simulink model "lab1dulepovMinina22017"  (R2017a)
settings: Solver=ode23tb  StartTime=0.0  StopTime=1  MaxStep=1e-4  RelTol=1e-5
undefined symbols (not defined in the file): load, source, transparam
libraries: powerlib x9, powerlib_meascontrol x3
settings Model: Creator=Student11  LastModifiedBy=админ
settings SolverCC: MaxConsecutiveMinStep=2
settings DebuggingCC: IgnoredZcDiagnostic=none  UnconnectedInputMsg=none  UnconnectedOutputMsg=none  UnconnectedLineMsg=none
settings SimscapeCC: SimscapeNormalizeSystem=off

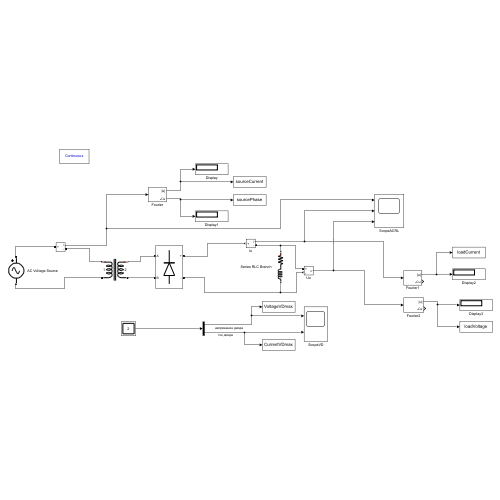
[thumbnail: Simulink's stored preview of the top-level diagram]
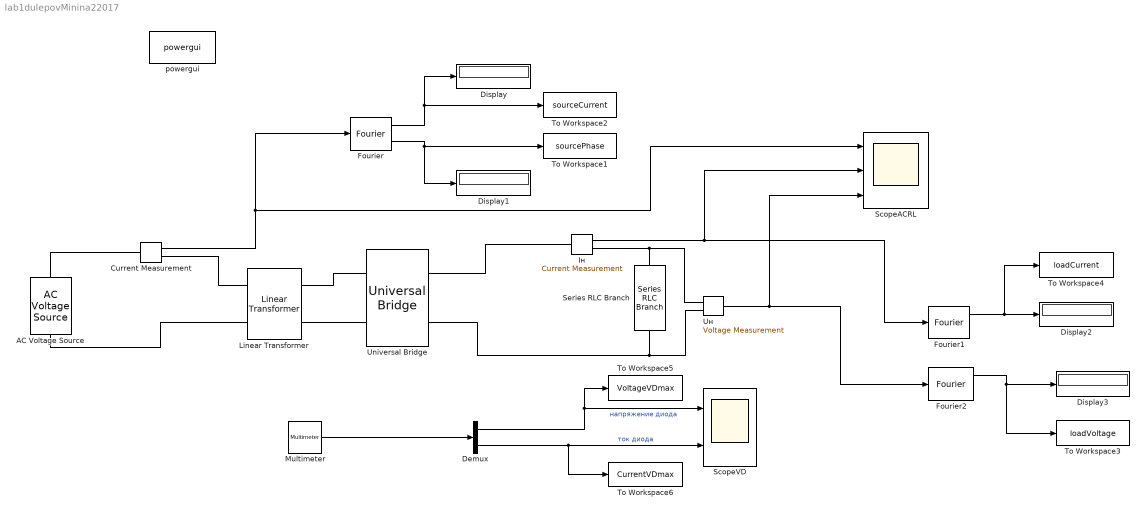
== system lab1dulepovMinina22017 ==
  AC Voltage Source : powerlib/Electrical Sources/AC Voltage Source  Amplitude=source.voltage  Phase=0  Frequency=source.freq  SampleTime=0  Measurements=None  BusType=swing  Pref=10e3  Qref=0  Qmin=-inf  Qmax=+inf
  Current Measurement : powerlib/Measurements/Current Measurement  PhasorSimulation=off  OutputType=Complex  PSBequivalent=0
  Demux : Demux  Outputs=2
  Display{,1..3} (4 alike) : Display
  Fourier : powerlib_meascontrol/Measurements/Fourier  Freq=source.freq  n=1  InInit=[0, 0]  Ts=0
  Fourier1 : powerlib_meascontrol/Measurements/Fourier  Freq=source.freq  n=0  InInit=[0, 0]  Ts=0
  Fourier2 : powerlib_meascontrol/Measurements/Fourier  Freq=source.freq  n=0  InInit=[0, 0]  Ts=0
  Iн : powerlib/Measurements/Current Measurement  PhasorSimulation=off  OutputType=Complex  PSBequivalent=0
  Linear Transformer : powerlib/Elements/Linear Transformer  UNITS=SI  NominalPower=[transparam.power source.freq]  winding1=[transparam.volt1wing 0.01 0.000001]  winding2=[transparam.volt2wing 0.04 0.000004]  ThreeWindings=off  winding3=[3.15e+05 992.25 63.169]  RmLm=[5000 5000]  Measurements=None  DataType=on
  Multimeter : powerlib/Measurements/Multimeter  L=10  sel=[1 7]  yselected={}  Gain=[1 1]  OutputType=Complex  PlotAtSimulationStop=off  PhasorSimulation=off
  ScopeVD : Scope  NumInputPorts=2
  ScopeАСRL : Scope  NumInputPorts=3
  Series RLC Branch : powerlib/Elements/Series RLC Branch  LConnTagsString=__new0  RConnTagsString=__new0  BranchType=RL  Resistance=load.Res  Inductance=load.Ind  SetiL0=off  InitialCurrent=0  Capacitance=1e-6  Setx0=off  InitialVoltage=0  Measurements=None
  To Workspace1 : ToWorkspace  VariableName=sourcePhase  SampleTime=-1
      settings: Save2DSignal=2-D array (concatenate along first dimension)
  To Workspace2 : ToWorkspace  VariableName=sourceCurrent  SampleTime=-1
      settings: Save2DSignal=2-D array (concatenate along first dimension)
  To Workspace3 : ToWorkspace  VariableName=loadVoltage  SampleTime=-1
      settings: Save2DSignal=2-D array (concatenate along first dimension)
  To Workspace4 : ToWorkspace  VariableName=loadCurrent  SampleTime=-1
      settings: Save2DSignal=2-D array (concatenate along first dimension)
  To Workspace5 : ToWorkspace  VariableName=VoltageVDmax  SampleTime=-1
      settings: Save2DSignal=2-D array (concatenate along first dimension)
  To Workspace6 : ToWorkspace  VariableName=CurrentVDmax  SampleTime=-1
      settings: Save2DSignal=2-D array (concatenate along first dimension)
  Universal Bridge : powerlib/Power Electronics/Universal Bridge  Arms=2  SnubberResistance=1e5  SnubberCapacitance=inf  Device=Diodes  Ron=1e-3  Lon=0  ForwardVoltages="[  0  0  ]"  ForwardVoltage=2  GTOparameters=[ 10e-6 , 20e-6 ]  IGBTparameters=[ 1e-6 , 2e-6 ]  Measurements=All voltages and currents  Measurements_2=None  converterType=Rectifier
  Uн : powerlib/Measurements/Voltage Measurement  PhasorSimulation=off  OutputType=Complex  PSBequivalent=0
  powergui : powerlib/powergui  Priority=1  SimulationMode=Continuous  SampleTime=50e-6  frequency=60  Iterations=50  frequencyindice=0  Pbase=100e6  ErrMax=1e-4  UnitsV=kV  UnitsW=MW  buscounter=0  FunctionMessages=off  echomessages=off  EnableUseOfTLC=off  CurrentSourceSwitches=off  DisableSnubberDevices=off  DisableRonSwitches=off  DisableVfSwitches=off  DisplayEquations=off  AutomaticDiscreteSolvers=off  SolverType=Tustin/Backward Euler (TBE)  Interpol=off  ExternalGateDelay=off  methode=off  Ts=100  x0status=blocks  SPID=on  SwTol=0  HookPort=off  NonlinearTolerance=1e-4  nMaxIteration=100  ContinueOnMaxIteration=off  RestoreLinks=warning  ResistiveCurrentMeasurement=off  Frange=[0:2:500]  Ylog=off  Xlog=on  ShowGrid=off  save=off  variable=ZData  structure=0  ZoomFFT=off  StartTime=0.0  cycles=1  DisplayStyle=1  fundamental=60  FreqAxis=off  MaxFrequency=1000  frequencyindicesteady=1  RmsSteady=1  display=off
  wires:
  Fourier/2 -> To Workspace1/1, Display1/1
  Fourier/1 -> To Workspace2/1, Display/1
  Uн/1 -> ScopeАСRL/3, Fourier2/1
  Fourier2/1 -> Display3/1, To Workspace3/1
  Fourier1/1 -> To Workspace4/1, Display2/1
  Current Measurement/1 -> ScopeАСRL/1, Fourier/1
  Iн/1 -> ScopeАСRL/2, Fourier1/1
  Demux/2 -> ScopeVD/2, To Workspace6/1  "ток диода"
  Demux/1 -> ScopeVD/1, To Workspace5/1  "напряжение диода"
  Multimeter/1 -> Demux/1
  connections:
  AC Voltage Source/RConn1 -- Current Measurement/LConn1
  Current Measurement/RConn1 -- Linear Transformer/LConn1
  Linear Transformer/LConn2 -- AC Voltage Source/LConn1
  Linear Transformer/RConn1 -- Universal Bridge/LConn1
  Linear Transformer/RConn2 -- Universal Bridge/LConn2
  Iн/LConn1 -- Universal Bridge/RConn1
  Iн/RConn1 -- Uн/LConn1 -- Series RLC Branch/LConn1
  Universal Bridge/RConn2 -- Uн/LConn2 -- Series RLC Branch/RConn1
